simulink model "gm_UZ_EnDat"  (R2023b)
settings: Solver=FixedStepDiscrete  StartTime=0  StopTime=0.002  RelTol=1e-3
model workspace (MAT data in the model file):
  Select = 0
libraries: hdlsllib x314, hdlmdlgenlib x10, simulink x7, simulink_extras x3
(part 3 of 7)

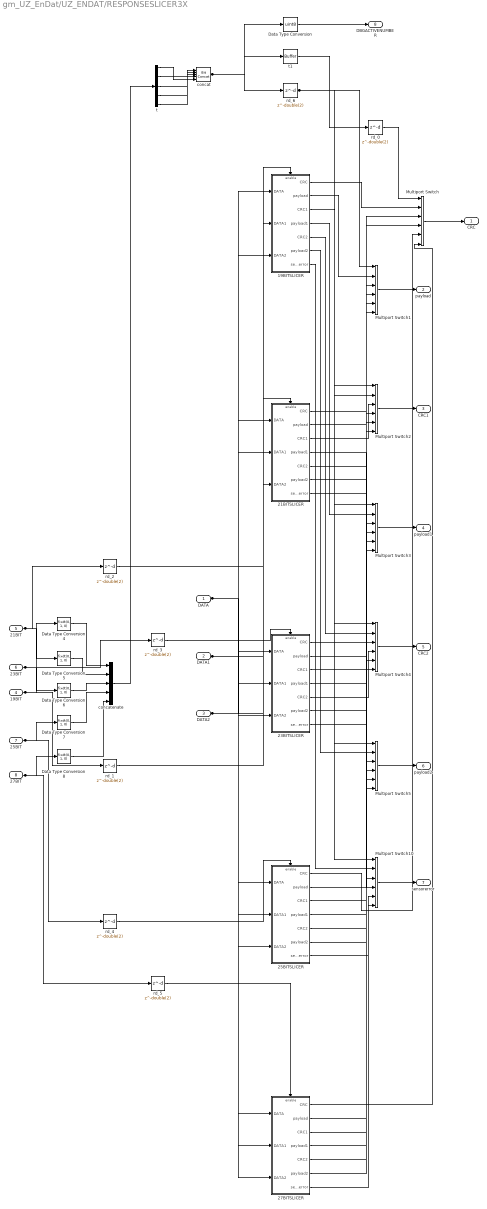
== system gm_UZ_EnDat/UZ_ENDAT/RESPONSESLICER3X ==
  DATA : Inport  OutDataTypeStr=fixdt(0, 64, 0)  PortDimensions=1  SampleTime=1e-08
  DATA1 : Inport  Port=2  OutDataTypeStr=fixdt(0, 64, 0)  PortDimensions=1  SampleTime=1e-08
  DATA2 : Inport  Port=3  OutDataTypeStr=fixdt(0, 64, 0)  PortDimensions=1  SampleTime=1e-08
  19BIT : Inport  Port=4  OutDataTypeStr=boolean  PortDimensions=1  SampleTime=1e-08
  21BIT : Inport  Port=5  OutDataTypeStr=boolean  PortDimensions=1  SampleTime=1e-08
  23BIT : Inport  Port=6  OutDataTypeStr=boolean  PortDimensions=1  SampleTime=1e-08
  25BIT : Inport  Port=7  OutDataTypeStr=boolean  PortDimensions=1  SampleTime=1e-08
  27BIT : Inport  Port=8  OutDataTypeStr=boolean  PortDimensions=1  SampleTime=1e-08
  19BITSLICER : Subsystem
  21BITSLICER : Subsystem
  23BITSLICER : Subsystem
  25BITSLICER : Subsystem
  27BITSLICER : Subsystem
  Data Type Conversion : DataTypeConversion  OutDataTypeStr=uint8  RndMeth=Nearest  SampleTime=1e-08  SaturateOnIntegerOverflow=off
  Data Type Conversion{4..8} (5 alike) : DataTypeConversion  OutDataTypeStr=fixdt(0, 1, 0)  SampleTime=1e-08  SaturateOnIntegerOverflow=off  RndMeth=Floor
  Multiport Switch : MultiPortSwitch  DataPortOrder=Specify indices  Inputs=5  DataPortIndices={ double(1) double(2) double(4) double(8) double(16)}  DiagnosticForDefault=None  OutDataTypeStr=uint8  RndMeth=Simplest  SampleTime=1e-08  SaturateOnIntegerOverflow=off  InputSameDT=off
  Multiport Switch1 : MultiPortSwitch  DataPortOrder=Specify indices  Inputs=5  DataPortIndices={ double(1) double(2) double(4) double(8) double(16)}  DiagnosticForDefault=None  OutDataTypeStr=uint32  RndMeth=Simplest  SampleTime=1e-08  SaturateOnIntegerOverflow=off  InputSameDT=off
  Multiport Switch10 : MultiPortSwitch  DataPortOrder=Specify indices  Inputs=5  DataPortIndices={ double(1) double(2) double(4) double(8) double(16)}  DiagnosticForDefault=None  RndMeth=Simplest  SampleTime=1e-08  SaturateOnIntegerOverflow=off  InputSameDT=off
  Multiport Switch2 : MultiPortSwitch  DataPortOrder=Specify indices  Inputs=5  DataPortIndices={ double(1) double(2) double(4) double(8) double(16)}  DiagnosticForDefault=None  OutDataTypeStr=uint8  RndMeth=Simplest  SampleTime=1e-08  SaturateOnIntegerOverflow=off  InputSameDT=off
  Multiport Switch3 : MultiPortSwitch  DataPortOrder=Specify indices  Inputs=5  DataPortIndices={ double(1) double(2) double(4) double(8) double(16)}  DiagnosticForDefault=None  OutDataTypeStr=uint32  RndMeth=Simplest  SampleTime=1e-08  SaturateOnIntegerOverflow=off  InputSameDT=off
  Multiport Switch4 : MultiPortSwitch  DataPortOrder=Specify indices  Inputs=5  DataPortIndices={ double(1) double(2) double(4) double(8) double(16)}  DiagnosticForDefault=None  OutDataTypeStr=uint8  RndMeth=Simplest  SampleTime=1e-08  SaturateOnIntegerOverflow=off  InputSameDT=off
  Multiport Switch5 : MultiPortSwitch  DataPortOrder=Specify indices  Inputs=5  DataPortIndices={ double(1) double(2) double(4) double(8) double(16)}  DiagnosticForDefault=None  OutDataTypeStr=uint32  RndMeth=Simplest  SampleTime=1e-08  SaturateOnIntegerOverflow=off  InputSameDT=off
  concat : hdlsllib/Logic and Bit Operations/Bit Concat  numInputs=5
  concatenate : Concatenate  NumInputs=5
  rd_{0..6} (7 alike) : Delay  DelayLength=double(2)  InitialCondition=0  SampleTime=1e-08
  t : Demux  Outputs=5
  t1 : hdlmdlgenlib/Buffer
  CRC : Outport  SampleTime=1e-08
  payload : Outport  Port=2  SampleTime=1e-08
  CRC1 : Outport  Port=3  SampleTime=1e-08
  payload1 : Outport  Port=4  SampleTime=1e-08
  CRC2 : Outport  Port=5  SampleTime=1e-08
  payload2 : Outport  Port=6  SampleTime=1e-08
  sensorerror : Outport  Port=7  OutDataTypeStr=boolean  SampleTime=1e-08
  DBGACTIVENUMBER : Outport  Port=8  SampleTime=1e-08
  wires:
  DATA/1 -> 19BITSLICER/1(DATA), 21BITSLICER/1(DATA), 23BITSLICER/1(DATA), 27BITSLICER/1(DATA), 25BITSLICER/1(DATA)
  DATA1/1 -> 19BITSLICER/2(DATA1), 21BITSLICER/2(DATA1), 23BITSLICER/2(DATA1), 27BITSLICER/2(DATA1), 25BITSLICER/2(DATA1)
  DATA2/1 -> 21BITSLICER/3(DATA2), 19BITSLICER/3(DATA2), 23BITSLICER/3(DATA2), 27BITSLICER/3(DATA2), 25BITSLICER/3(DATA2)
  19BITSLICER/1(CRC) -> Multiport Switch/2
  19BITSLICER/2(payload) -> Multiport Switch1/2
  19BITSLICER/3(CRC1) -> Multiport Switch2/2
  19BITSLICER/4(payload1) -> Multiport Switch3/2
  19BITSLICER/5(CRC2) -> Multiport Switch4/2
  19BITSLICER/6(payload2) -> Multiport Switch5/2
  19BITSLICER/7(sensorerror) -> Multiport Switch10/2
  21BITSLICER/1(CRC) -> Multiport Switch/3
  21BITSLICER/2(payload) -> Multiport Switch1/3
  21BITSLICER/3(CRC1) -> Multiport Switch2/3
  21BITSLICER/4(payload1) -> Multiport Switch3/3
  21BITSLICER/5(CRC2) -> Multiport Switch4/3
  21BITSLICER/6(payload2) -> Multiport Switch5/3
  21BITSLICER/7(sensorerror) -> Multiport Switch10/3
  23BITSLICER/1(CRC) -> Multiport Switch/4
  23BITSLICER/2(payload) -> Multiport Switch1/4
  23BITSLICER/3(CRC1) -> Multiport Switch2/4
  23BITSLICER/4(payload1) -> Multiport Switch3/4
  23BITSLICER/5(CRC2) -> Multiport Switch4/4
  23BITSLICER/6(payload2) -> Multiport Switch5/4
  23BITSLICER/7(sensorerror) -> Multiport Switch10/4
  25BITSLICER/1(CRC) -> Multiport Switch/5
  25BITSLICER/2(payload) -> Multiport Switch1/5
  25BITSLICER/3(CRC1) -> Multiport Switch2/5
  25BITSLICER/4(payload1) -> Multiport Switch3/5
  25BITSLICER/5(CRC2) -> Multiport Switch4/5
  25BITSLICER/6(payload2) -> Multiport Switch5/5
  25BITSLICER/7(sensorerror) -> Multiport Switch10/5
  27BITSLICER/1(CRC) -> Multiport Switch/6
  27BITSLICER/2(payload) -> Multiport Switch1/6
  27BITSLICER/3(CRC1) -> Multiport Switch2/6
  27BITSLICER/4(payload1) -> Multiport Switch3/6
  27BITSLICER/5(CRC2) -> Multiport Switch4/6
  27BITSLICER/6(payload2) -> Multiport Switch5/6
  27BITSLICER/7(sensorerror) -> Multiport Switch10/6
  t1/1 -> rd_0/1
  Data Type Conversion/1 -> DBGACTIVENUMBER/1
  Data Type Conversion4/1 -> concatenate/1
  Data Type Conversion5/1 -> concatenate/2
  Data Type Conversion6/1 -> concatenate/3
  Data Type Conversion7/1 -> concatenate/4
  Data Type Conversion8/1 -> concatenate/5
  Multiport Switch/1 -> CRC/1
  Multiport Switch1/1 -> payload/1
  Multiport Switch10/1 -> sensorerror/1
  Multiport Switch2/1 -> CRC1/1
  Multiport Switch3/1 -> payload1/1
  Multiport Switch4/1 -> CRC2/1
  Multiport Switch5/1 -> payload2/1
  concatenate/1 -> t/1
  t/1 -> concat/5
  t/2 -> concat/4
  t/3 -> concat/3
  t/4 -> concat/2
  t/5 -> concat/1
  19BIT/1 -> rd_1/1, Data Type Conversion4/1
  21BIT/1 -> rd_2/1, Data Type Conversion5/1
  23BIT/1 -> rd_3/1, Data Type Conversion6/1
  25BIT/1 -> rd_4/1, Data Type Conversion7/1
  27BIT/1 -> rd_5/1, Data Type Conversion8/1
  rd_5/1 -> 27BITSLICER/Enable
  rd_2/1 -> 21BITSLICER/Enable
  rd_3/1 -> 23BITSLICER/Enable
  rd_4/1 -> 25BITSLICER/Enable
  rd_1/1 -> 19BITSLICER/Enable
  rd_0/1 -> Multiport Switch/1
  concat/1 -> t1/1, Data Type Conversion/1, rd_6/1
  rd_6/1 -> Multiport Switch1/1, Multiport Switch3/1, Multiport Switch5/1, Multiport Switch2/1, Multiport Switch4/1, Multiport Switch10/1

== system gm_UZ_EnDat/UZ_ENDAT/SetZeroBool ==
  valin : Inport  OutDataTypeStr=boolean  PortDimensions=1
  setzero : Inport  Port=2  OutDataTypeStr=boolean  PortDimensions=1
  Trigger : TriggerPort  TriggerType=either  VariantControl=(inherit)  PortDimensions=1  OutDataTypeStr=boolean
  Constant1 : Constant  OutDataTypeStr=boolean  SampleTime=-1
  Constant2 : Constant  Value=0  OutDataTypeStr=boolean  SampleTime=-1
  Index Vector1 : MultiPortSwitch  DataPortOrder=Zero-based contiguous  Inputs=2  DiagnosticForDefault=None  zeroidx=on  SaturateOnIntegerOverflow=off  InputSameDT=off
  Logical Operator : Logic  AllPortsSameDT=off  OutDataTypeStr=boolean
  valueout : Outport  InitialOutput=0  VectorParamsAs1DForOutWhenUnconnected=off
  wires:
  valin/1 -> Logical Operator/2
  setzero/1 -> Index Vector1/1
  Constant1/1 -> Index Vector1/2
  Constant2/1 -> Index Vector1/3
  Index Vector1/1 -> Logical Operator/1
  Logical Operator/1 -> valueout/1

== system gm_UZ_EnDat/UZ_ENDAT/SetZeroBool1 ==
  valin : Inport  OutDataTypeStr=boolean  PortDimensions=1
  setzero : Inport  Port=2  OutDataTypeStr=boolean  PortDimensions=1
  Trigger : TriggerPort  TriggerType=either  VariantControl=(inherit)  PortDimensions=1  OutDataTypeStr=boolean
  Constant1 : Constant  OutDataTypeStr=boolean  SampleTime=-1
  Constant2 : Constant  Value=0  OutDataTypeStr=boolean  SampleTime=-1
  Index Vector1 : MultiPortSwitch  DataPortOrder=Zero-based contiguous  Inputs=2  DiagnosticForDefault=None  zeroidx=on  SaturateOnIntegerOverflow=off  InputSameDT=off
  Logical Operator : Logic  AllPortsSameDT=off  OutDataTypeStr=boolean
  valueout : Outport  InitialOutput=0  VectorParamsAs1DForOutWhenUnconnected=off
  wires:
  valin/1 -> Logical Operator/2
  setzero/1 -> Index Vector1/1
  Constant1/1 -> Index Vector1/2
  Constant2/1 -> Index Vector1/3
  Index Vector1/1 -> Logical Operator/1
  Logical Operator/1 -> valueout/1

== system gm_UZ_EnDat/UZ_ENDAT/SetZeroBool2 ==
  valin : Inport  OutDataTypeStr=boolean  PortDimensions=1
  setzero : Inport  Port=2  OutDataTypeStr=boolean  PortDimensions=1
  Trigger : TriggerPort  TriggerType=either  VariantControl=(inherit)  PortDimensions=1  OutDataTypeStr=boolean
  Constant1 : Constant  OutDataTypeStr=boolean  SampleTime=-1
  Constant2 : Constant  Value=0  OutDataTypeStr=boolean  SampleTime=-1
  Index Vector1 : MultiPortSwitch  DataPortOrder=Zero-based contiguous  Inputs=2  DiagnosticForDefault=None  zeroidx=on  SaturateOnIntegerOverflow=off  InputSameDT=off
  Logical Operator : Logic  AllPortsSameDT=off  OutDataTypeStr=boolean
  valueout : Outport  InitialOutput=0  VectorParamsAs1DForOutWhenUnconnected=off
  wires:
  valin/1 -> Logical Operator/2
  setzero/1 -> Index Vector1/1
  Constant1/1 -> Index Vector1/2
  Constant2/1 -> Index Vector1/3
  Index Vector1/1 -> Logical Operator/1
  Logical Operator/1 -> valueout/1

== system gm_UZ_EnDat/UZ_ENDAT/SetZeroBool3 ==
  valin : Inport  OutDataTypeStr=boolean  PortDimensions=1
  setzero : Inport  Port=2  OutDataTypeStr=boolean  PortDimensions=1
  Trigger : TriggerPort  TriggerType=either  VariantControl=(inherit)  PortDimensions=1  OutDataTypeStr=boolean
  Constant1 : Constant  OutDataTypeStr=boolean  SampleTime=-1
  Constant2 : Constant  Value=0  OutDataTypeStr=boolean  SampleTime=-1
  Index Vector1 : MultiPortSwitch  DataPortOrder=Zero-based contiguous  Inputs=2  DiagnosticForDefault=None  zeroidx=on  SaturateOnIntegerOverflow=off  InputSameDT=off
  Logical Operator : Logic  AllPortsSameDT=off  OutDataTypeStr=boolean
  valueout : Outport  InitialOutput=0  VectorParamsAs1DForOutWhenUnconnected=off
  wires:
  valin/1 -> Logical Operator/2
  setzero/1 -> Index Vector1/1
  Constant1/1 -> Index Vector1/2
  Constant2/1 -> Index Vector1/3
  Index Vector1/1 -> Logical Operator/1
  Logical Operator/1 -> valueout/1

== system gm_UZ_EnDat/UZ_ENDAT/SetZeroBool4 ==
  valin : Inport  OutDataTypeStr=boolean  PortDimensions=1
  setzero : Inport  Port=2  OutDataTypeStr=boolean  PortDimensions=1
  Trigger : TriggerPort  TriggerType=either  VariantControl=(inherit)  PortDimensions=1  OutDataTypeStr=boolean
  Constant1 : Constant  OutDataTypeStr=boolean  SampleTime=-1
  Constant2 : Constant  Value=0  OutDataTypeStr=boolean  SampleTime=-1
  Index Vector1 : MultiPortSwitch  DataPortOrder=Zero-based contiguous  Inputs=2  DiagnosticForDefault=None  zeroidx=on  SaturateOnIntegerOverflow=off  InputSameDT=off
  Logical Operator : Logic  AllPortsSameDT=off  OutDataTypeStr=boolean
  valueout : Outport  InitialOutput=0  VectorParamsAs1DForOutWhenUnconnected=off
  wires:
  valin/1 -> Logical Operator/2
  setzero/1 -> Index Vector1/1
  Constant1/1 -> Index Vector1/2
  Constant2/1 -> Index Vector1/3
  Index Vector1/1 -> Logical Operator/1
  Logical Operator/1 -> valueout/1

== system gm_UZ_EnDat/UZ_ENDAT/SetZeroBool5 ==
  valin : Inport  OutDataTypeStr=boolean  PortDimensions=1
  setzero : Inport  Port=2  OutDataTypeStr=boolean  PortDimensions=1
  Trigger : TriggerPort  TriggerType=either  VariantControl=(inherit)  PortDimensions=1  OutDataTypeStr=boolean
  Constant1 : Constant  OutDataTypeStr=boolean  SampleTime=-1
  Constant2 : Constant  Value=0  OutDataTypeStr=boolean  SampleTime=-1
  Index Vector1 : MultiPortSwitch  DataPortOrder=Zero-based contiguous  Inputs=2  DiagnosticForDefault=None  zeroidx=on  SaturateOnIntegerOverflow=off  InputSameDT=off
  Logical Operator : Logic  AllPortsSameDT=off  OutDataTypeStr=boolean
  valueout : Outport  InitialOutput=0  VectorParamsAs1DForOutWhenUnconnected=off
  wires:
  valin/1 -> Logical Operator/2
  setzero/1 -> Index Vector1/1
  Constant1/1 -> Index Vector1/2
  Constant2/1 -> Index Vector1/3
  Index Vector1/1 -> Logical Operator/1
  Logical Operator/1 -> valueout/1

== system gm_UZ_EnDat/UZ_ENDAT/Storage16 ==
  Data : Inport  OutDataTypeStr=uint16  PortDimensions=1  SampleTime=1e-08
  Write : Inport  Port=2  OutDataTypeStr=boolean  PortDimensions=1  SampleTime=1e-08
  Compare To Zero : Subsystem  mask(Compare To Zero){relop===, OutDataTypeStr=boolean, ZeroCross=on}
      mask prompts: relop "Simulink:masks:Operator_MP"; OutDataTypeStr "Simulink:masks:OutputDataType_MP"; ZeroCross "Simulink:masks:EnableZerocrossingDetection_MP"
      mask help: Simulink:masks:CompareToZero_MD
      mask init:
      | OutDataTypeStr = 'boolean';
      | ZeroCross = 'on';
      | blkName = 'UZ_EnDat/UZ_ENDAT/Storage16/Compare\nTo Zero';
      | relop = '==';
      | setValue = 'boolean';
      mask TypeOptions relop: == | ~= | < | <= | >= | >
      mask TypeOptions OutDataTypeStr: Simulink:masks:uint8 | Simulink:masks:boolean
      mask Callback ZeroCross: sl('zeroCrossEnable', gcbh);
      mask Display: disp([relop,' 0'])
  Logical Operator : Logic  Operator=NOT  Inputs=1  AllPortsSameDT=off  OutDataTypeStr=boolean  SampleTime=1e-08
  Logical Operator1 : Logic  Inputs=3  AllPortsSameDT=off  OutDataTypeStr=boolean  SampleTime=1e-08
  Logical Operator2 : Logic  Operator=NOT  Inputs=1  AllPortsSameDT=off  OutDataTypeStr=boolean  SampleTime=1e-08
  Logical Operator3 : Logic  AllPortsSameDT=off  OutDataTypeStr=boolean  SampleTime=1e-08
  Relational Operator : RelationalOperator  Operator===  OutDataTypeStr=boolean  SampleTime=1e-08  InputSameDT=off
  Single Port RAM System : hdlsllib/HDL RAMs/Single Port RAM System  RAMType=Single port  AsyncRead=off  WriteOutputValue=Old data  RAMInitialValue=0  allowBusInputs=off  WritesHaveOutput=on  NumReads=0  NumWrites=1  SimulateUsing=Code generation
  adress : Constant  Value=5  OutDataTypeStr=uint8  SampleTime=1e-08
  out : Outport  SampleTime=1e-08
  wrok : Outport  Port=2  OutDataTypeStr=boolean  SampleTime=1e-08
  wires:
  Data/1 -> Compare To Zero/1(u), Relational Operator/2, Single Port RAM System/1
  Write/1 -> Logical Operator1/1
  Compare To Zero/1(y) -> Logical Operator2/1
  Logical Operator2/1 -> Logical Operator3/2, Logical Operator1/3
  Logical Operator3/1 -> wrok/1
  Relational Operator/1 -> Logical Operator3/1, Logical Operator/1
  Single Port RAM System/1 -> out/1, Relational Operator/1
  adress/1 -> Single Port RAM System/2
  Logical Operator/1 -> Logical Operator1/2
  Logical Operator1/1 -> Single Port RAM System/3

== system gm_UZ_EnDat/UZ_ENDAT/Subsystem ==
  CLK : Inport  OutDataTypeStr=boolean  PortDimensions=1  SampleTime=1e-08
  RESET : Inport  Port=2  OutDataTypeStr=boolean  PortDimensions=1  SampleTime=1e-08
  CLKS2DATAFLOWCHG : Inport  Port=3  OutDataTypeStr=uint8  PortDimensions=1  SampleTime=1e-08
  CLK2ENDOFTRANSMISSION : Inport  Port=4  OutDataTypeStr=uint16  PortDimensions=1  SampleTime=1e-08
  VERYSLOWCLK : Inport  Port=5  OutDataTypeStr=boolean  PortDimensions=1  SampleTime=1e-08
  Constant : Constant  OutDataTypeStr=boolean  SampleTime=1e-08
  Constant1 : Constant  Value=0  OutDataTypeStr=boolean  SampleTime=1e-08
  CLKOUT : Outport  SampleTime=1e-08
  DATAOUT : Outport  Port=2  SampleTime=1e-08
  BOOTUPCOMPLETE : Outport  Port=3  SampleTime=1e-08
  DATAINV : Outport  Port=4  SampleTime=1e-08
  wires:
  Constant/1 -> DATAINV/1, BOOTUPCOMPLETE/1, CLKOUT/1
  Constant1/1 -> DATAOUT/1

== system gm_UZ_EnDat/UZ_ENDAT/Subsystem1 ==
  in : Inport  OutDataTypeStr=fixdt(0, 1, 0)  PortDimensions=[5]  SampleTime=1e-08
  Enable : EnablePort  OutDataTypeStr=boolean
  concat : hdlsllib/Logic and Bit Operations/Bit Concat  numInputs=5
  t : Demux  Outputs=5
  out : Outport  SampleTime=1e-08  InitialOutput=0
  wires:
  in/1 -> t/1
  concat/1 -> out/1
  t/1 -> concat/5
  t/2 -> concat/4
  t/3 -> concat/3
  t/4 -> concat/2
  t/5 -> concat/1

== system gm_UZ_EnDat/UZ_ENDAT/Subsystem2 ==
  CLK : Inport  OutDataTypeStr=boolean  PortDimensions=1  SampleTime=1e-08
  SLOWCLCK : Inport  Port=2  OutDataTypeStr=boolean  PortDimensions=1  SampleTime=1e-08
  DATA : Inport  Port=3  OutDataTypeStr=uint16  PortDimensions=1  SampleTime=1e-08
  reset : Inport  Port=4  OutDataTypeStr=boolean  PortDimensions=1  SampleTime=1e-08
  Enable : EnablePort  OutDataTypeStr=boolean
  ManualDeserializere : Subsystem
  valin : Outport  SampleTime=1e-08  InitialOutput=0
  wires:
  CLK/1 -> ManualDeserializere/1(CLK)
  SLOWCLCK/1 -> ManualDeserializere/2(SLOWCLCK)
  DATA/1 -> ManualDeserializere/3(DATA)
  reset/1 -> ManualDeserializere/4(reset)
  ManualDeserializere/1(valin) -> valin/1

== system gm_UZ_EnDat/UZ_ENDAT/Subsystem6 ==
  In1 : Inport  OutDataTypeStr=uint16  PortDimensions=1  SampleTime=1e-08
  FACTOR : Inport  Port=2  OutMin=0  OutMax=60000  OutDataTypeStr=uint16  PortDimensions=1  SampleTime=1e-08
  Constant : Constant  Value=100  OutDataTypeStr=uint16  SampleTime=1e-08
  Divide : Product  Inputs=*/  OutDataTypeStr=uint16  RndMeth=Simplest  SaturateOnIntegerOverflow=on  SampleTime=1e-08
  HwModeRegister : Delay  DelayLength=double(1)  InitialCondition=0  SampleTime=1e-08
  HwModeRegister1 : Delay  DelayLength=double(1)  InitialCondition=0  SampleTime=1e-08
  PipelineRegister : Delay  DelayLength=double(1)  InitialCondition=0  SampleTime=1e-08
  Product : Product  Inputs=**  OutDataTypeStr=uint32  SampleTime=1e-08
  Product_out_dtc : DataTypeConversion  OutDataTypeStr=uint16  RndMeth=Simplest  SampleTime=1e-08
  Out1 : Outport  SampleTime=1e-08
  wires:
  In1/1 -> HwModeRegister/1
  FACTOR/1 -> HwModeRegister1/1
  Constant/1 -> Divide/2
  Divide/1 -> Out1/1
  Product_out_dtc/1 -> Divide/1
  PipelineRegister/1 -> Product_out_dtc/1
  Product/1 -> PipelineRegister/1
  HwModeRegister/1 -> Product/1
  HwModeRegister1/1 -> Product/2

== system gm_UZ_EnDat/UZ_ENDAT/ageprovider ==
  wrok : Inport  OutDataTypeStr=boolean  PortDimensions=1  SampleTime=1e-08
  recieving : Inport  Port=2  OutDataTypeStr=boolean  PortDimensions=1  SampleTime=1e-08
  altmode : Inport  Port=3  OutDataTypeStr=boolean  PortDimensions=1  SampleTime=1e-08
  Constant : Constant  Value=10  OutDataTypeStr=uint32  SampleTime=1e-08
  Detect Increase1 : Subsystem  mask(Detect Increase){vinit=double(0), InputProcessing=Elements as channels (sample based), OutDataTypeStr=boolean}
      mask prompts: vinit "Simulink:masks:InitialCondition_MP"; InputProcessing "Simulink:masks:InputProcessing_MP"; OutDataTypeStr "Simulink:masks:OutputDataType_MP"
      mask help: Simulink:masks:DetectIncrease_MD
      mask TypeOptions InputProcessing: Simulink:masks:ColumnsAsChannelsFrameBased | Simulink:masks:ElementsAsChannelsSampleBased
      mask TypeOptions OutDataTypeStr: Simulink:masks:uint8 | Simulink:masks:boolean
      mask Display: fprintf('U > U/z')
  HDL Counter_enbsw : Switch  Criteria=u2 ~= 0  Threshold=double(0)  OutDataTypeStr=uint32  SampleTime=1e-08  SaturateOnIntegerOverflow=off  InputSameDT=off
  HwModeRegister : Delay  DelayLength=double(1)  InitialCondition=0  SampleTime=1e-08
  HwModeRegister1 : Delay  DelayLength=double(1)  InitialCondition=0  SampleTime=1e-08
  Logical Operator1 : Logic  Operator=NOT  Inputs=1  AllPortsSameDT=off  OutDataTypeStr=boolean  SampleTime=1e-08
  PipelineRegister : Delay  DelayLength=double(1)  InitialCondition=0  SampleTime=1e-08
  Switch : Switch  Criteria=u2 ~= 0  Threshold=double(0)  OutDataTypeStr=boolean  SampleTime=1e-08  SaturateOnIntegerOverflow=off  InputSameDT=off
  adder : Sum  OutDataTypeStr=uint32  AccumDataTypeStr=uint32  SampleTime=1e-08
  const : Constant  Value=0  VectorParams1D=off  OutDataTypeStr=uint32  SampleTime=1e-08
  nsproduct : Product  Inputs=**  OutDataTypeStr=fixdt(0, 64, 0)  SampleTime=1e-08
  nsproduct_out_dtc : DataTypeConversion  OutDataTypeStr=uint32  RndMeth=Simplest  SampleTime=1e-08
  rd_0 : Delay  DelayLength=double(2)  InitialCondition=0  SampleTime=1e-08
  rd_1 : Delay  DelayLength=double(2)  InitialCondition=0  SampleTime=1e-08
  rd_2 : Delay  DelayLength=double(1)  InitialCondition=0  SampleTime=1e-08
  stateControl : Constant  OutDataTypeStr=boolean  SampleTime=1e-08
  step_value : Constant  VectorParams1D=off  OutDataTypeStr=uint32  SampleTime=1e-08
  switchEnable : MultiPortSwitch  DataPortOrder=Zero-based contiguous  Inputs=2  DiagnosticForDefault=None  zeroidx=on  OutDataTypeStr=uint32  SampleTime=1e-08  SaturateOnIntegerOverflow=off  InputSameDT=off
  switchReset : Switch  Criteria=u2 ~= 0  Threshold=double(0)  OutDataTypeStr=uint32  SampleTime=1e-08  SaturateOnIntegerOverflow=off  InputSameDT=off
  posage : Outport  OutDataTypeStr=uint32  SampleTime=1e-08
  wires:
  wrok/1 -> Switch/3
  recieving/1 -> Switch/1
  Constant/1 -> HwModeRegister/1
  Detect Increase1/1(Y) -> Logical Operator1/1, switchReset/2
  Switch/1 -> Detect Increase1/1(U)
  nsproduct_out_dtc/1 -> posage/1
  PipelineRegister/1 -> nsproduct_out_dtc/1
  altmode/1 -> rd_0/1
  stateControl/1 -> rd_1/1
  step_value/1 -> adder/2
  Logical Operator1/1 -> switchEnable/1
  const/1 -> switchReset/1
  adder/1 -> switchEnable/3
  switchEnable/1 -> switchReset/3
  switchReset/1 -> HDL Counter_enbsw/1
  rd_1/1 -> HDL Counter_enbsw/2
  rd_0/1 -> Switch/2
  HDL Counter_enbsw/1 -> rd_2/1
  rd_2/1 -> HDL Counter_enbsw/3, adder/1, switchEnable/2, HwModeRegister1/1
  nsproduct/1 -> PipelineRegister/1
  HwModeRegister/1 -> nsproduct/1
  HwModeRegister1/1 -> nsproduct/2

== system gm_UZ_EnDat/UZ_ENDAT/ramselektor ==
  In1 : Inport  OutMin=0  OutMax=15  OutDataTypeStr=fixdt(0, 4, 0)  PortDimensions=1  LockScale=on
  Trigger : TriggerPort  VariantControl=(inherit)  OutputDataType=int8  InitialTriggerSignalState=positive  PortDimensions=1  OutDataTypeStr=boolean
  Delay : Delay  DelayLength=double(99)  InitialCondition=0
  Increment Stored Integer : Subsystem  mask(Stored Integer Value Increment){}
      mask help: Simulink:masks:StoredIntegerValueIncrement_MD
      mask Display: disp('Q++')
  SEL : Outport  InitialOutput=0
  wires:
  Delay/1 -> Increment Stored Integer/1(u)
  Increment Stored Integer/1(y) -> SEL/1
  In1/1 -> Delay/1

== system gm_UZ_EnDat/UZ_ENDAT/signalquality ==
  wrok : Inport  OutDataTypeStr=boolean  PortDimensions=1  SampleTime=1e-08
  Detect Increase1 : Subsystem  mask(Detect Increase){vinit=double(0), InputProcessing=Elements as channels (sample based), OutDataTypeStr=boolean}
      mask prompts: vinit "Simulink:masks:InitialCondition_MP"; InputProcessing "Simulink:masks:InputProcessing_MP"; OutDataTypeStr "Simulink:masks:OutputDataType_MP"
      mask help: Simulink:masks:DetectIncrease_MD
      mask TypeOptions InputProcessing: Simulink:masks:ColumnsAsChannelsFrameBased | Simulink:masks:ElementsAsChannelsSampleBased
      mask TypeOptions OutDataTypeStr: Simulink:masks:uint8 | Simulink:masks:boolean
      mask Display: fprintf('U > U/z')
  HDL Counter1_enbsw : Switch  Criteria=u2 ~= 0  Threshold=double(0)  OutDataTypeStr=uint16  SampleTime=1e-08  SaturateOnIntegerOverflow=off  InputSameDT=off
  Memory_enbsw : Switch  Criteria=u2 ~= 0  Threshold=double(0)  OutDataTypeStr=uint16  SampleTime=1e-08  SaturateOnIntegerOverflow=off  InputSameDT=off
  Switch1 : Switch  Criteria=u2 ~= 0  Threshold=double(0)  OutDataTypeStr=uint16  SampleTime=1e-08  SaturateOnIntegerOverflow=off  InputSameDT=off
  adder : Sum  OutDataTypeStr=uint32  AccumDataTypeStr=uint32  SampleTime=1e-08
  adder1 : Sum  OutDataTypeStr=uint16  AccumDataTypeStr=uint16  SampleTime=1e-08
  compare : simulink/Logic and Bit Operations/Compare To Constant  relop=>  const="fi(0,0,32,0,\"hex\",\"fffffffe\")"  OutDataTypeStr=boolean
  compare1 : simulink/Logic and Bit Operations/Compare To Constant  relop===  const="fi(0,0,32,0,\"hex\",\"05f5e100\")"  OutDataTypeStr=boolean
  const : Constant  Value=0  VectorParams1D=off  OutDataTypeStr=uint16  SampleTime=1e-08
  countFrom : Constant  Value=0  VectorParams1D=off  OutDataTypeStr=uint32  SampleTime=1e-08
  or : Logic  Operator=OR  AllPortsSameDT=off  OutDataTypeStr=boolean  SampleTime=1e-08
  rd_0 : Delay  DelayLength=double(1)  InitialCondition=0  SampleTime=1e-08
  rd_1 : Delay  DelayLength=double(2)  InitialCondition=0  SampleTime=1e-08
  rd_2 : Delay  DelayLength=double(2)  InitialCondition=0  SampleTime=1e-08
  rd_3 : Delay  DelayLength=double(1)  InitialCondition=0  SampleTime=1e-08
  rd_4 : Delay  DelayLength=double(2)  InitialCondition=0  SampleTime=1e-08
  rd_5 : Delay  DelayLength=double(1)  InitialCondition=0  SampleTime=1e-08
  stateControl : Constant  OutDataTypeStr=boolean  SampleTime=1e-08
  stateControl1 : Constant  OutDataTypeStr=boolean  SampleTime=1e-08
  step_value : Constant  VectorParams1D=off  OutDataTypeStr=uint32  SampleTime=1e-08
  step_value1 : Constant  VectorParams1D=off  OutDataTypeStr=uint16  SampleTime=1e-08
  switch : Switch  Criteria=u2 ~= 0  Threshold=double(0)  OutDataTypeStr=uint32  SampleTime=1e-08  SaturateOnIntegerOverflow=off  InputSameDT=off
  switchEnable : MultiPortSwitch  DataPortOrder=Zero-based contiguous  Inputs=2  DiagnosticForDefault=None  zeroidx=on  OutDataTypeStr=uint16  SampleTime=1e-08  SaturateOnIntegerOverflow=off  InputSameDT=off
  switchReset : Switch  Criteria=u2 ~= 0  Threshold=double(0)  OutDataTypeStr=uint16  SampleTime=1e-08  SaturateOnIntegerOverflow=off  InputSameDT=off
  amoundofsyncs : Outport  OutDataTypeStr=uint16  SampleTime=1e-08
  wires:
  wrok/1 -> Detect Increase1/1(U)
  compare1/1 -> or/1, switch/2
  compare/1 -> or/2
  stateControl/1 -> rd_2/1
  stateControl1/1 -> rd_4/1
  Switch1/1 -> Memory_enbsw/1, amoundofsyncs/1
  step_value/1 -> adder/2
  countFrom/1 -> switch/1
  adder/1 -> switch/3
  step_value1/1 -> adder1/2
  Detect Increase1/1(Y) -> switchEnable/1
  const/1 -> switchReset/1
  adder1/1 -> switchEnable/3
  switchEnable/1 -> switchReset/3
  switchReset/1 -> HDL Counter1_enbsw/1
  rd_2/1 -> HDL Counter1_enbsw/2
  rd_4/1 -> Memory_enbsw/2
  or/1 -> rd_1/1
  rd_1/1 -> Switch1/2, switchReset/2
  switch/1 -> rd_0/1
  rd_0/1 -> compare/1, adder/1, compare1/1
  HDL Counter1_enbsw/1 -> rd_3/1
  rd_3/1 -> HDL Counter1_enbsw/3, adder1/1, switchEnable/2, Switch1/1
  Memory_enbsw/1 -> rd_5/1
  rd_5/1 -> Memory_enbsw/3, Switch1/3

== system gm_UZ_EnDat/UZ_ENDAT/timingprovider ==
  wrok : Inport  OutDataTypeStr=boolean  PortDimensions=1  SampleTime=1e-08
  clk : Inport  Port=2  OutDataTypeStr=boolean  PortDimensions=1  SampleTime=1e-08
  CLKCNTER_POSCNTR : Subsystem
  CLKCNTER_POSCNTR1 : Subsystem
  Compare To Constant : Subsystem  mask(Compare To Constant){relop=>, const=double(3), OutDataTypeStr=boolean, ZeroCross=on}
      mask prompts: relop "Simulink:masks:Operator_MP"; const "Simulink:masks:ConstantValue_MP"; OutDataTypeStr "Simulink:masks:OutputDataType_MP"; ZeroCross "Simulink:masks:EnableZerocrossingDetection_MP"
      mask help: Simulink:masks:CompareToConstant_MD
      mask TypeOptions relop: == | ~= | < | <= | >= | >
      mask TypeOptions OutDataTypeStr: Simulink:masks:uint8 | Simulink:masks:boolean
      mask Callback ZeroCross: sl('zeroCrossEnable', gcbh);
      mask Display: disp(str)
  Compare To Constant1 : Subsystem  mask(Compare To Constant){relop===, const=double(0), OutDataTypeStr=boolean, ZeroCross=on}
      mask prompts: relop "Simulink:masks:Operator_MP"; const "Simulink:masks:ConstantValue_MP"; OutDataTypeStr "Simulink:masks:OutputDataType_MP"; ZeroCross "Simulink:masks:EnableZerocrossingDetection_MP"
      mask help: Simulink:masks:CompareToConstant_MD
      mask TypeOptions relop: == | ~= | < | <= | >= | >
      mask TypeOptions OutDataTypeStr: Simulink:masks:uint8 | Simulink:masks:boolean
      mask Callback ZeroCross: sl('zeroCrossEnable', gcbh);
      mask Display: disp(str)
  Detect Increase1 : Subsystem  mask(Detect Increase){vinit=double(0), InputProcessing=Elements as channels (sample based), OutDataTypeStr=boolean}
      mask prompts: vinit "Simulink:masks:InitialCondition_MP"; InputProcessing "Simulink:masks:InputProcessing_MP"; OutDataTypeStr "Simulink:masks:OutputDataType_MP"
      mask help: Simulink:masks:DetectIncrease_MD
      mask TypeOptions InputProcessing: Simulink:masks:ColumnsAsChannelsFrameBased | Simulink:masks:ElementsAsChannelsSampleBased
      mask TypeOptions OutDataTypeStr: Simulink:masks:uint8 | Simulink:masks:boolean
      mask Display: fprintf('U > U/z')
  Logical Operator : Logic  Operator=OR  AllPortsSameDT=off  OutDataTypeStr=boolean  SampleTime=1e-08
  Subsystem2 : Subsystem
  Subsystem3 : Subsystem
  rd_0 : Delay  DelayLength=double(2)  InitialCondition=0  SampleTime=1e-08
  rd_1 : Delay  DelayLength=double(2)  InitialCondition=0  SampleTime=1e-08
  timeelapsed2cycl : Outport  OutDataTypeStr=uint32  SampleTime=1e-08
  timeelapsed1cycl : Outport  Port=2  OutDataTypeStr=uint32  SampleTime=1e-08
  wires:
  wrok/1 -> Detect Increase1/1(U)
  CLKCNTER_POSCNTR/1(CNT) -> Subsystem3/2(clkcnt), Subsystem2/2(clkcnt)
  CLKCNTER_POSCNTR1/1(CNT) -> Subsystem3/1(elapsed), Subsystem2/1(elapsed), Compare To Constant/1(u), Compare To Constant1/1(u)
  Compare To Constant1/1(y) -> Logical Operator/2
  Detect Increase1/1(Y) -> CLKCNTER_POSCNTR1/2(CLK2CNT)
  Logical Operator/1 -> CLKCNTER_POSCNTR/3(ResetCNT)
  Subsystem2/1(ns elapsed) -> timeelapsed2cycl/1
  Subsystem3/1(ns elapsed) -> timeelapsed1cycl/1
  clk/1 -> rd_0/1, CLKCNTER_POSCNTR/2(CLK2CNT), CLKCNTER_POSCNTR/1(CLK)
  rd_0/1 -> CLKCNTER_POSCNTR1/1(CLK)
  Compare To Constant/1(y) -> rd_1/1
  rd_1/1 -> CLKCNTER_POSCNTR1/3(ResetCNT), Logical Operator/1

== system gm_UZ_EnDat/UZ_ENDAT/3timestorage/Compare To Constant ==
  u : Inport  OutDataTypeStr=uint8  SampleTime=1e-08
  Compare : RelationalOperator  Operator===  OutDataTypeStr=boolean  SampleTime=1e-08
  Constant : Constant  Value=0  OutDataTypeStr=uint8  SampleTime=1e-08
  y : Outport  SampleTime=1e-08
  wires:
  u/1 -> Compare/1
  Compare/1 -> y/1
  Constant/1 -> Compare/2

== system gm_UZ_EnDat/UZ_ENDAT/3timestorage/Compare To Constant1 ==
  u : Inport  OutDataTypeStr=uint8  SampleTime=1e-08
  Compare : RelationalOperator  Operator===  OutDataTypeStr=boolean
  Constant : Constant  DisableCoverage=on  Value=const  OutDataTypeStr=Inherit: Inherit via back propagation  SampleTime=-1
  y : Outport  SampleTime=1e-08
  wires:
  u/1 -> Compare/1
  Compare/1 -> y/1
  Constant/1 -> Compare/2

== system gm_UZ_EnDat/UZ_ENDAT/3timestorage/Compare To Constant2 ==
  u : Inport  OutDataTypeStr=uint8  SampleTime=1e-08
  Compare : RelationalOperator  Operator===  OutDataTypeStr=boolean
  Constant : Constant  DisableCoverage=on  Value=const  OutDataTypeStr=Inherit: Inherit via back propagation  SampleTime=-1
  y : Outport  SampleTime=1e-08
  wires:
  u/1 -> Compare/1
  Compare/1 -> y/1
  Constant/1 -> Compare/2

== system gm_UZ_EnDat/UZ_ENDAT/3timestorage/Detect Increase2 ==
  note: U(k)
  note: Edge
  U : Inport  OutDataTypeStr=boolean  SampleTime=1e-08
  FixPt Relational Operator : RelationalOperator  Operator=>  OutDataTypeStr=boolean  SampleTime=1e-08  InputSameDT=off
  rd_0 : Delay  DelayLength=double(1)  InitialCondition=0  SampleTime=1e-08
  t : hdlmdlgenlib/Buffer
  Y : Outport  SampleTime=1e-08
  wires:
  U/1 -> t/1, FixPt Relational Operator/1
  t/1 -> rd_0/1
  FixPt Relational Operator/1 -> Y/1
  rd_0/1 -> FixPt Relational Operator/2

== system gm_UZ_EnDat/UZ_ENDAT/3timestorage/Detect Increase3 ==
  note: U(k)
  note: Edge
  U : Inport  OutDataTypeStr=boolean  SampleTime=1e-08
  FixPt Relational Operator : RelationalOperator  Operator=>  OutDataTypeStr=boolean  SampleTime=1e-08  InputSameDT=off
  rd_0 : Delay  DelayLength=double(1)  InitialCondition=0  SampleTime=1e-08
  t : hdlmdlgenlib/Buffer
  Y : Outport  SampleTime=1e-08
  wires:
  U/1 -> t/1, FixPt Relational Operator/1
  t/1 -> rd_0/1
  FixPt Relational Operator/1 -> Y/1
  rd_0/1 -> FixPt Relational Operator/2

== system gm_UZ_EnDat/UZ_ENDAT/3timestorage/Detect Increase4 ==
  note: U(k)
  note: Edge
  U : Inport  OutDataTypeStr=boolean  SampleTime=1e-08
  FixPt Relational Operator : RelationalOperator  Operator=>  OutDataTypeStr=boolean  SampleTime=1e-08  InputSameDT=off
  rd_0 : Delay  DelayLength=double(1)  InitialCondition=0  SampleTime=1e-08
  t : hdlmdlgenlib/Buffer
  Y : Outport  SampleTime=1e-08
  wires:
  U/1 -> t/1, FixPt Relational Operator/1
  t/1 -> rd_0/1
  FixPt Relational Operator/1 -> Y/1
  rd_0/1 -> FixPt Relational Operator/2

== system gm_UZ_EnDat/UZ_ENDAT/3timestorage/Storage1 ==
  Data : Inport  OutDataTypeStr=fixdt(0, 64, 0)  PortDimensions=1  SampleTime=1e-08
  Write : Inport  Port=2  OutDataTypeStr=boolean  PortDimensions=1  SampleTime=1e-08
  Delay2 : Delay  DelayLength=double(1)  InitialCondition=0  SampleTime=1e-08
  Switch : Switch  Criteria=u2 > Threshold  Threshold=double(0)  OutDataTypeStr=fixdt(0, 64, 0)  SampleTime=1e-08  SaturateOnIntegerOverflow=off  InputSameDT=off
  out : Outport  SampleTime=1e-08
  wires:
  Switch/1 -> out/1, Delay2/1
  Data/1 -> Switch/1
  Write/1 -> Switch/2
  Delay2/1 -> Switch/3

== system gm_UZ_EnDat/UZ_ENDAT/3timestorage/Storage2 ==
  Data : Inport  OutDataTypeStr=fixdt(0, 64, 0)  PortDimensions=1  SampleTime=1e-08
  Write : Inport  Port=2  OutDataTypeStr=boolean  PortDimensions=1  SampleTime=1e-08
  Delay2 : Delay  DelayLength=double(1)  InitialCondition=0  SampleTime=1e-08
  Switch : Switch  Criteria=u2 > Threshold  Threshold=double(0)  OutDataTypeStr=fixdt(0, 64, 0)  SampleTime=1e-08  SaturateOnIntegerOverflow=off  InputSameDT=off
  out : Outport  SampleTime=1e-08
  wires:
  Delay2/1 -> Switch/3
  Write/1 -> Switch/2
  Data/1 -> Switch/1
  Switch/1 -> Delay2/1, out/1

== system gm_UZ_EnDat/UZ_ENDAT/3timestorage/Storage20 ==
  Data : Inport  OutDataTypeStr=fixdt(0, 64, 0)  PortDimensions=1  SampleTime=1e-08
  Write : Inport  Port=2  OutDataTypeStr=boolean  PortDimensions=1  SampleTime=1e-08
  Delay2 : Delay  DelayLength=double(1)  InitialCondition=0  SampleTime=1e-08
  Switch : Switch  Criteria=u2 > Threshold  Threshold=double(0)  OutDataTypeStr=fixdt(0, 64, 0)  SampleTime=1e-08  SaturateOnIntegerOverflow=off  InputSameDT=off
  out : Outport  SampleTime=1e-08
  wires:
  Delay2/1 -> Switch/3
  Write/1 -> Switch/2
  Data/1 -> Switch/1
  Switch/1 -> Delay2/1, out/1

== system gm_UZ_EnDat/UZ_ENDAT/3timestorage/Triggered Subsystem ==
  Trigger : TriggerPort  VariantControl=(inherit)  PortDimensions=1  OutDataTypeStr=boolean
  Counter Limited : Subsystem  mask(Counter Limited){uplimit=double(2), tsamp=double(-1)}
      mask prompts: uplimit "Simulink:masks:UpperLimit_MP"; tsamp "Simulink:masks:SampleTime_MP"
      mask help: Simulink:masks:CounterLimited_MD
  Out1 : Outport  InitialOutput=0
  wires:
  Counter Limited/1(y) -> Out1/1

== system gm_UZ_EnDat/UZ_ENDAT/8BIT_SPLITTER/Compare To Constant ==
  u : Inport  OutDataTypeStr=fixdt(0, 4, 0)
  Compare : RelationalOperator  Operator===  OutDataTypeStr=boolean
  Constant : Constant  Value=0  OutDataTypeStr=fixdt(0, 4, 0)  SampleTime=-1
  y : Outport  InitialOutput=0
  wires:
  u/1 -> Compare/1
  Compare/1 -> y/1
  Constant/1 -> Compare/2

== system gm_UZ_EnDat/UZ_ENDAT/8BIT_SPLITTER/Compare To Constant1 ==
  u : Inport  OutDataTypeStr=fixdt(0, 4, 0)
  Compare : RelationalOperator  Operator===  OutDataTypeStr=boolean
  Constant : Constant  DisableCoverage=on  Value=const  OutDataTypeStr=Inherit: Inherit via back propagation  SampleTime=-1
  y : Outport  InitialOutput=0
  wires:
  u/1 -> Compare/1
  Compare/1 -> y/1
  Constant/1 -> Compare/2

== system gm_UZ_EnDat/UZ_ENDAT/8BIT_SPLITTER/Compare To Constant2 ==
  u : Inport  OutDataTypeStr=fixdt(0, 4, 0)
  Compare : RelationalOperator  Operator===  OutDataTypeStr=boolean
  Constant : Constant  DisableCoverage=on  Value=const  OutDataTypeStr=Inherit: Inherit via back propagation  SampleTime=-1
  y : Outport  InitialOutput=0
  wires:
  u/1 -> Compare/1
  Compare/1 -> y/1
  Constant/1 -> Compare/2

== system gm_UZ_EnDat/UZ_ENDAT/8BIT_SPLITTER/Compare To Constant3 ==
  u : Inport  OutDataTypeStr=fixdt(0, 4, 0)
  Compare : RelationalOperator  Operator===  OutDataTypeStr=boolean
  Constant : Constant  DisableCoverage=on  Value=const  OutDataTypeStr=Inherit: Inherit via back propagation  SampleTime=-1
  y : Outport  InitialOutput=0
  wires:
  u/1 -> Compare/1
  Compare/1 -> y/1
  Constant/1 -> Compare/2

== system gm_UZ_EnDat/UZ_ENDAT/8BIT_SPLITTER/Compare To Constant4 ==
  u : Inport  OutDataTypeStr=fixdt(0, 4, 0)
  Compare : RelationalOperator  Operator===  OutDataTypeStr=boolean
  Constant : Constant  DisableCoverage=on  Value=const  OutDataTypeStr=Inherit: Inherit via back propagation  SampleTime=-1
  y : Outport  InitialOutput=0
  wires:
  u/1 -> Compare/1
  Compare/1 -> y/1
  Constant/1 -> Compare/2

== system gm_UZ_EnDat/UZ_ENDAT/8BIT_SPLITTER/Compare To Constant5 ==
  u : Inport  OutDataTypeStr=fixdt(0, 4, 0)
  Compare : RelationalOperator  Operator===  OutDataTypeStr=boolean
  Constant : Constant  DisableCoverage=on  Value=const  OutDataTypeStr=Inherit: Inherit via back propagation  SampleTime=-1
  y : Outport  InitialOutput=0
  wires:
  u/1 -> Compare/1
  Compare/1 -> y/1
  Constant/1 -> Compare/2

== system gm_UZ_EnDat/UZ_ENDAT/8BIT_SPLITTER/Compare To Constant6 ==
  u : Inport  OutDataTypeStr=fixdt(0, 4, 0)
  Compare : RelationalOperator  Operator===  OutDataTypeStr=boolean
  Constant : Constant  DisableCoverage=on  Value=const  OutDataTypeStr=Inherit: Inherit via back propagation  SampleTime=-1
  y : Outport  InitialOutput=0
  wires:
  u/1 -> Compare/1
  Compare/1 -> y/1
  Constant/1 -> Compare/2

== system gm_UZ_EnDat/UZ_ENDAT/8BIT_SPLITTER/Compare To Constant7 ==
  u : Inport  OutDataTypeStr=fixdt(0, 4, 0)
  Compare : RelationalOperator  Operator===  OutDataTypeStr=boolean
  Constant : Constant  DisableCoverage=on  Value=const  OutDataTypeStr=Inherit: Inherit via back propagation  SampleTime=-1
  y : Outport  InitialOutput=0
  wires:
  u/1 -> Compare/1
  Compare/1 -> y/1
  Constant/1 -> Compare/2

== system gm_UZ_EnDat/UZ_ENDAT/CLKCNTER_ACT/Positional_Counter ==
  valueout : Inport  OutDataTypeStr=uint32  PortDimensions=1
  Trigger : TriggerPort  VariantControl=(inherit)  InitialTriggerSignalState=zero  PortDimensions=1  OutDataTypeStr=boolean
  Increment Stored Integer : Subsystem  mask(Stored Integer Value Increment){}
      mask help: Simulink:masks:StoredIntegerValueIncrement_MD
      mask Display: disp('Q++')
  divider : Outport  InitialOutput=0
  wires:
  Increment Stored Integer/1(y) -> divider/1
  valueout/1 -> Increment Stored Integer/1(u)

== system gm_UZ_EnDat/UZ_ENDAT/CLKCNTER_ACT/SetZero32modified ==
  valin : Inport  OutDataTypeStr=uint32  PortDimensions=1
  setzero : Inport  Port=2  OutDataTypeStr=boolean  PortDimensions=1
  Trigger : TriggerPort  TriggerType=either  VariantControl=(inherit)  PortDimensions=1  OutDataTypeStr=boolean
  Constant2 : Constant  Value=0  OutDataTypeStr=uint32  SampleTime=-1
  Index Vector1 : MultiPortSwitch  DataPortOrder=Zero-based contiguous  Inputs=2  DiagnosticForDefault=None  zeroidx=on  OutDataTypeStr=uint32  SaturateOnIntegerOverflow=off  InputSameDT=off
  valueout : Outport  InitialOutput=0  VectorParamsAs1DForOutWhenUnconnected=off
  wires:
  Index Vector1/1 -> valueout/1
  Constant2/1 -> Index Vector1/3
  setzero/1 -> Index Vector1/1
  valin/1 -> Index Vector1/2

== system gm_UZ_EnDat/UZ_ENDAT/CLKCNTER_NOSTOP/Positional_Counter ==
  valueout : Inport  OutDataTypeStr=uint32  PortDimensions=1
  Trigger : TriggerPort  VariantControl=(inherit)  InitialTriggerSignalState=zero  PortDimensions=1  OutDataTypeStr=boolean
  Increment Stored Integer : Subsystem  mask(Stored Integer Value Increment){}
      mask help: Simulink:masks:StoredIntegerValueIncrement_MD
      mask Display: disp('Q++')
  divider : Outport  InitialOutput=0
  wires:
  valueout/1 -> Increment Stored Integer/1(u)
  Increment Stored Integer/1(y) -> divider/1

== system gm_UZ_EnDat/UZ_ENDAT/CLKCNTER_NOSTOP/SetZero32modified ==
  valin : Inport  OutDataTypeStr=uint32  PortDimensions=1
  setzero : Inport  Port=2  OutDataTypeStr=boolean  PortDimensions=1
  Trigger : TriggerPort  TriggerType=either  VariantControl=(inherit)  PortDimensions=1  OutDataTypeStr=boolean
  Constant2 : Constant  Value=0  OutDataTypeStr=uint32  SampleTime=-1
  Index Vector1 : MultiPortSwitch  DataPortOrder=Zero-based contiguous  Inputs=2  DiagnosticForDefault=None  zeroidx=on  OutDataTypeStr=uint32  SaturateOnIntegerOverflow=off  InputSameDT=off
  valueout : Outport  InitialOutput=0  VectorParamsAs1DForOutWhenUnconnected=off
  wires:
  valin/1 -> Index Vector1/2
  setzero/1 -> Index Vector1/1
  Constant2/1 -> Index Vector1/3
  Index Vector1/1 -> valueout/1

== system gm_UZ_EnDat/UZ_ENDAT/CLKDIV1/Triggered Subsystem ==
  IN : Inport  OutDataTypeStr=boolean  PortDimensions=1
  Trigger : TriggerPort  VariantControl=(inherit)  OutputDataType=int8  InitialTriggerSignalState=positive  PortDimensions=1  OutDataTypeStr=boolean
  OUT : Outport  InitialOutput=0
  wires:
  IN/1 -> OUT/1

== system gm_UZ_EnDat/UZ_ENDAT/CLKDIV3/Triggered Subsystem ==
  IN : Inport  OutDataTypeStr=boolean  PortDimensions=1
  Trigger : TriggerPort  VariantControl=(inherit)  OutputDataType=int8  InitialTriggerSignalState=positive  PortDimensions=1  OutDataTypeStr=boolean
  OUT : Outport  InitialOutput=0
  wires:
  IN/1 -> OUT/1

== system gm_UZ_EnDat/UZ_ENDAT/CLKDIV4/Triggered Subsystem ==
  IN : Inport  OutDataTypeStr=boolean  PortDimensions=1
  Trigger : TriggerPort  VariantControl=(inherit)  OutputDataType=int8  InitialTriggerSignalState=positive  PortDimensions=1  OutDataTypeStr=boolean
  OUT : Outport  InitialOutput=0
  wires:
  IN/1 -> OUT/1

== system gm_UZ_EnDat/UZ_ENDAT/CLKDIV5/Triggered Subsystem ==
  IN : Inport  OutDataTypeStr=boolean  PortDimensions=1
  Trigger : TriggerPort  VariantControl=(inherit)  OutputDataType=int8  InitialTriggerSignalState=positive  PortDimensions=1  OutDataTypeStr=boolean
  OUT : Outport  InitialOutput=0
  wires:
  IN/1 -> OUT/1

== system gm_UZ_EnDat/UZ_ENDAT/CLKDIV6/Triggered Subsystem ==
  IN : Inport  OutDataTypeStr=boolean  PortDimensions=1
  Trigger : TriggerPort  VariantControl=(inherit)  OutputDataType=int8  InitialTriggerSignalState=positive  PortDimensions=1  OutDataTypeStr=boolean
  OUT : Outport  InitialOutput=0
  wires:
  IN/1 -> OUT/1

== system gm_UZ_EnDat/UZ_ENDAT/CLKDIV7/Triggered Subsystem ==
  IN : Inport  OutDataTypeStr=boolean  PortDimensions=1
  Trigger : TriggerPort  VariantControl=(inherit)  OutputDataType=int8  InitialTriggerSignalState=positive  PortDimensions=1  OutDataTypeStr=boolean
  OUT : Outport  InitialOutput=0
  wires:
  IN/1 -> OUT/1

== system gm_UZ_EnDat/UZ_ENDAT/CLKDIV8/Triggered Subsystem ==
  IN : Inport  OutDataTypeStr=boolean  PortDimensions=1
  Trigger : TriggerPort  VariantControl=(inherit)  OutputDataType=int8  InitialTriggerSignalState=positive  PortDimensions=1  OutDataTypeStr=boolean
  OUT : Outport  InitialOutput=0
  wires:
  IN/1 -> OUT/1

== system gm_UZ_EnDat/UZ_ENDAT/CLKDIV9/Triggered Subsystem ==
  IN : Inport  OutDataTypeStr=boolean  PortDimensions=1
  Trigger : TriggerPort  VariantControl=(inherit)  OutputDataType=int8  InitialTriggerSignalState=positive  PortDimensions=1  OutDataTypeStr=boolean
  OUT : Outport  InitialOutput=0
  wires:
  IN/1 -> OUT/1

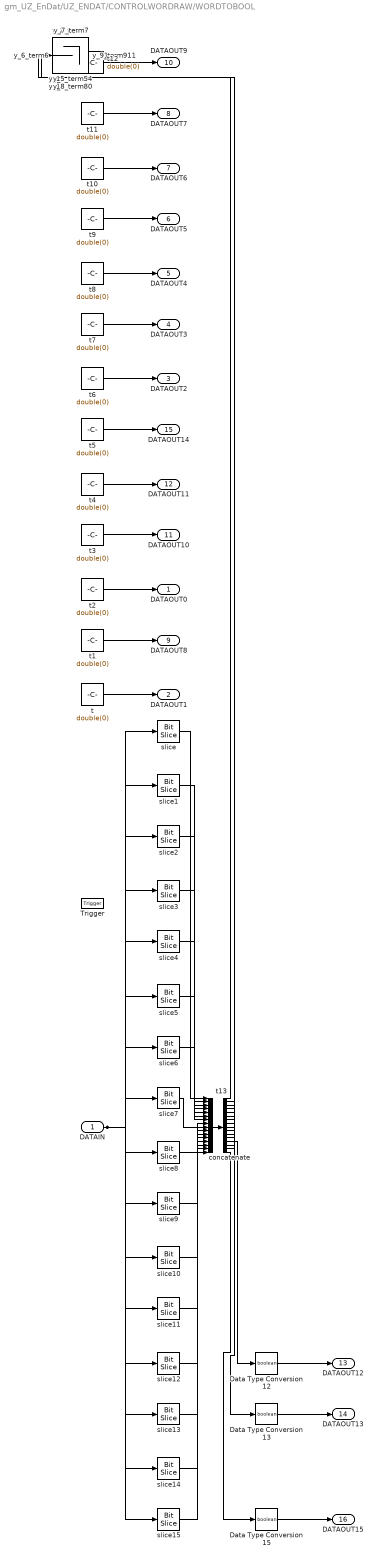
== system gm_UZ_EnDat/UZ_ENDAT/CONTROLWORDRAW/WORDTOBOOL ==
  DATAIN : Inport  OutDataTypeStr=uint16  PortDimensions=1
  Trigger : TriggerPort  TriggerType=falling  VariantControl=(inherit)  OutputDataType=int8  InitialTriggerSignalState=positive  PortDimensions=1  OutDataTypeStr=boolean
  Data Type Conversion12 : DataTypeConversion  OutDataTypeStr=boolean  SaturateOnIntegerOverflow=off  RndMeth=Floor
  Data Type Conversion13 : DataTypeConversion  OutDataTypeStr=boolean  SaturateOnIntegerOverflow=off  RndMeth=Floor
  Data Type Conversion15 : DataTypeConversion  OutDataTypeStr=boolean  SaturateOnIntegerOverflow=off  RndMeth=Floor
  concatenate : Concatenate  NumInputs=16  Mode=Multidimensional array  ConcatenateDimension=2
  slice : hdlsllib/Logic and Bit Operations/Bit Slice  lidx=double(0)  ridx=double(0)
  slice1 : hdlsllib/Logic and Bit Operations/Bit Slice  lidx=double(1)  ridx=double(1)
  slice10 : hdlsllib/Logic and Bit Operations/Bit Slice  lidx=double(10)  ridx=double(10)
  slice11 : hdlsllib/Logic and Bit Operations/Bit Slice  lidx=double(11)  ridx=double(11)
  slice12 : hdlsllib/Logic and Bit Operations/Bit Slice  lidx=double(12)  ridx=double(12)
  slice13 : hdlsllib/Logic and Bit Operations/Bit Slice  lidx=double(13)  ridx=double(13)
  slice14 : hdlsllib/Logic and Bit Operations/Bit Slice  lidx=double(14)  ridx=double(14)
  slice15 : hdlsllib/Logic and Bit Operations/Bit Slice  lidx=double(15)  ridx=double(15)
  slice2 : hdlsllib/Logic and Bit Operations/Bit Slice  lidx=double(2)  ridx=double(2)
  slice3 : hdlsllib/Logic and Bit Operations/Bit Slice  lidx=double(3)  ridx=double(3)
  slice4 : hdlsllib/Logic and Bit Operations/Bit Slice  lidx=double(4)  ridx=double(4)
  slice5 : hdlsllib/Logic and Bit Operations/Bit Slice  lidx=double(5)  ridx=double(5)
  slice6 : hdlsllib/Logic and Bit Operations/Bit Slice  lidx=double(6)  ridx=double(6)
  slice7 : hdlsllib/Logic and Bit Operations/Bit Slice  lidx=double(7)  ridx=double(7)
  slice8 : hdlsllib/Logic and Bit Operations/Bit Slice  lidx=double(8)  ridx=double(8)
  slice9 : hdlsllib/Logic and Bit Operations/Bit Slice  lidx=double(9)  ridx=double(9)
  t{,1..12} (13 alike) : Constant  Value=double(0)  OutDataTypeStr=boolean  SampleTime=-1
  t13 : Demux  Outputs=16
  y_0_term0 : Terminator
  y_10_term10 : Terminator
  y_11_term11 : Terminator
  y_14_term14 : Terminator
  y_1_term1 : Terminator
  y_2_term2 : Terminator
  y_3_term3 : Terminator
  y_4_term4 : Terminator
  y_5_term5 : Terminator
  y_6_term6 : Terminator
  y_7_term7 : Terminator
  y_8_term8 : Terminator
  y_9_term9 : Terminator
  DATAOUT0 : Outport  InitialOutput=0
  DATAOUT1 : Outport  Port=2  InitialOutput=0
  DATAOUT2 : Outport  Port=3  InitialOutput=0
  DATAOUT3 : Outport  Port=4  InitialOutput=0
  DATAOUT4 : Outport  Port=5  InitialOutput=0
  DATAOUT5 : Outport  Port=6  InitialOutput=0
  DATAOUT6 : Outport  Port=7  InitialOutput=0
  DATAOUT7 : Outport  Port=8  InitialOutput=0
  DATAOUT8 : Outport  Port=9  InitialOutput=0
  DATAOUT9 : Outport  Port=10  InitialOutput=0
  DATAOUT10 : Outport  Port=11  InitialOutput=0
  DATAOUT11 : Outport  Port=12  InitialOutput=0
  DATAOUT12 : Outport  Port=13  InitialOutput=0
  DATAOUT13 : Outport  Port=14  InitialOutput=0
  DATAOUT14 : Outport  Port=15  InitialOutput=0
  DATAOUT15 : Outport  Port=16  InitialOutput=0
  wires:
  DATAIN/1 -> slice15/1, slice14/1, slice13/1, slice12/1, slice11/1, slice10/1, slice9/1, slice8/1, slice7/1, slice6/1, slice5/1, slice4/1, slice3/1, slice2/1, slice1/1, slice/1
  t2/1 -> DATAOUT0/1
  t/1 -> DATAOUT1/1
  t3/1 -> DATAOUT10/1
  t4/1 -> DATAOUT11/1
  Data Type Conversion12/1 -> DATAOUT12/1
  Data Type Conversion13/1 -> DATAOUT13/1
  t5/1 -> DATAOUT14/1
  Data Type Conversion15/1 -> DATAOUT15/1
  t6/1 -> DATAOUT2/1
  t7/1 -> DATAOUT3/1
  t8/1 -> DATAOUT4/1
  t9/1 -> DATAOUT5/1
  t10/1 -> DATAOUT6/1
  t11/1 -> DATAOUT7/1
  t1/1 -> DATAOUT8/1
  t12/1 -> DATAOUT9/1
  concatenate/1 -> t13/1
  t13/1 -> y_0_term0/1
  t13/2 -> y_1_term1/1
  t13/3 -> y_2_term2/1
  t13/4 -> y_3_term3/1
  t13/5 -> y_4_term4/1
  t13/6 -> y_5_term5/1
  t13/7 -> y_6_term6/1
  t13/8 -> y_7_term7/1
  t13/9 -> y_8_term8/1
  t13/10 -> y_9_term9/1
  t13/11 -> y_10_term10/1
  t13/12 -> y_11_term11/1
  t13/13 -> Data Type Conversion12/1
  t13/14 -> Data Type Conversion13/1
  t13/15 -> y_14_term14/1
  t13/16 -> Data Type Conversion15/1
  slice/1 -> concatenate/1
  slice1/1 -> concatenate/2
  slice2/1 -> concatenate/3
  slice3/1 -> concatenate/4
  slice4/1 -> concatenate/5
  slice5/1 -> concatenate/6
  slice6/1 -> concatenate/7
  slice7/1 -> concatenate/8
  slice8/1 -> concatenate/9
  slice9/1 -> concatenate/10
  slice10/1 -> concatenate/11
  slice11/1 -> concatenate/12
  slice12/1 -> concatenate/13
  slice13/1 -> concatenate/14
  slice14/1 -> concatenate/15
  slice15/1 -> concatenate/16
